simulink model "PSOCDerate"  (R2024b)
settings: Solver=FixedStepAuto  StartTime=0.0  StopTime=10.0  RelTol=1e-3  EnableMultiTasking=on
settings Model: DataDictionary=Master_Dictionary.sldd  EnableAccessToBaseWorkspace=off  Creator=torni  LastModifiedBy=Will
settings OptimizationCC: DefaultParameterBehavior=Inlined  EnhancedBackFolding=on  PassReuseOutputArgsAs=Individual arguments  ZeroExternalMemoryAtStartup=off  ZeroInternalMemoryAtStartup=off  MaxStackSize=8192  OptimizeBlockOrder=speed  DifferentSizesBufferReuse=on  OptimizationCustomize=off  EfficientTunableParamExpr=on
settings DebuggingCC: ParameterTunabilityLossMsg=error
settings HardwareCC: ProdBitPerPointer=32  ProdBitPerSizeT=32  ProdBitPerPtrDiffT=32  ProdLargestAtomicInteger=Long  ProdLargestAtomicFloat=Double  ProdWordSize=32  ProdLongLongMode=on  ProdHWDeviceType=ARM Compatible->ARM Cortex-M
settings SFSimCC: MATLABDynamicMemAlloc=off
settings RTWCC: Description=Embedded Coder  SystemTargetFile=ert.tlc  HardwareBoard=STM32H7xx Based (Single-core)  TemplateMakefile=ert_default_tmf  Toolchain=GNU Tools for ARM Embedded Processors
settings CodeAppCC: ForceParamTrailComments=on  IgnoreCustomStorageClasses=off  OperatorAnnotations=on  SimulinkDataObjDesc=on  SFDataObjDesc=on  InsertBlockDesc=on
settings ERTTargetCC: TargetLangStandard=C99 (ISO)  CodeReplacementLibrary=ARM Cortex-M  ExtModeTransport=3  ExtModeStaticAlloc=on  ExtModeStaticAllocSize=2048  ExtModeMexFile=ext_xcp  ExtModeIntrfLevel=Level2 - Open

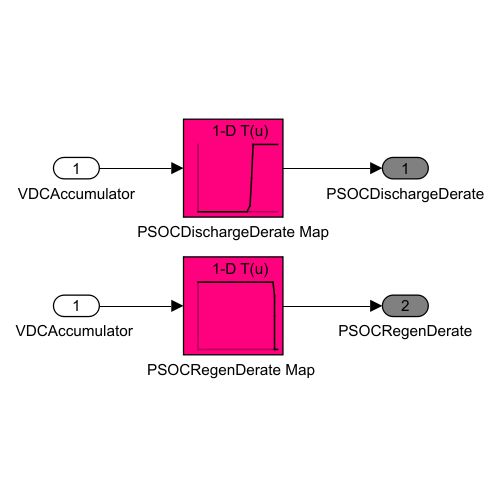
[thumbnail: Simulink's stored preview of the top-level diagram]
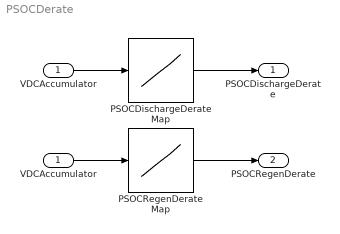
== system PSOCDerate ==
  VDCAccumulator : Inport  OutDataTypeStr=double
  PSOCDischargeDerate Map : Lookup_n-D  NumberOfTableDimensions=1  BreakpointsForDimension1=[0,377,390,403,416,600]  Table=[0,0,7.8,39,78,78]  InternalRulePriority=Speed  RndMeth=Simplest
  "PSOCRegenDerate Map " : Lookup_n-D  NumberOfTableDimensions=1  BreakpointsForDimension1=[0,569,574,576,578,600]  Table=[100,100,80,50,0,0]  InternalRulePriority=Speed  RndMeth=Simplest
  "VDCAccumulator " : InportShadow  OutDataTypeStr=double
  PSOCDischargeDerate : Outport  OutDataTypeStr=double  VectorParamsAs1DForOutWhenUnconnected=off
  PSOCRegenDerate : Outport  Port=2  OutDataTypeStr=double  VectorParamsAs1DForOutWhenUnconnected=off
  wires:
  VDCAccumulator/1 -> PSOCDischargeDerate Map/1
  PSOCDischargeDerate Map/1 -> PSOCDischargeDerate/1
  "PSOCRegenDerate Map "/1 -> PSOCRegenDerate/1
  "VDCAccumulator "/1 -> "PSOCRegenDerate Map "/1
